simulink model "HW4_Q2"  (R2023a)
settings: Solver=FixedStepAuto  StartTime=0.0  StopTime=10.0  FixedStep=0.001  RelTol=1e-3
values from neighbouring files (symbols this model uses):
  F0 = 1    [HW4_Q2_Script.m]    (also in HW4_Q3.m)
  k = 10    [HW4_Q2_Script.m]    (also in HW4_Q3.m)
  m = 1    [HW4_Q2_Script.m]    (also in HW4_Q3.m)
settings Model: Creator=DELL  LastModifiedBy=DELL
settings SolverCC: ZeroCrossAlgorithm=Adaptive
settings DebuggingCC: IgnoredZcDiagnostic=none

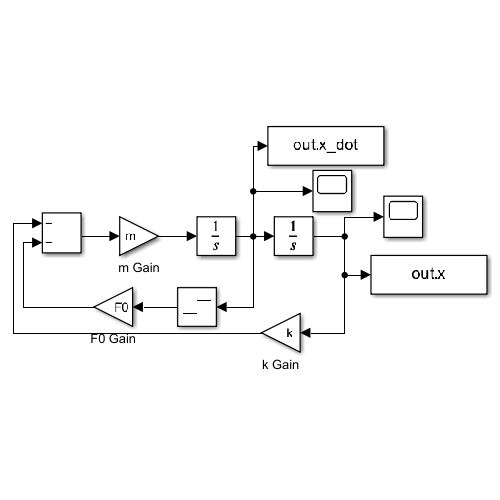
[thumbnail: Simulink's stored preview of the top-level diagram]
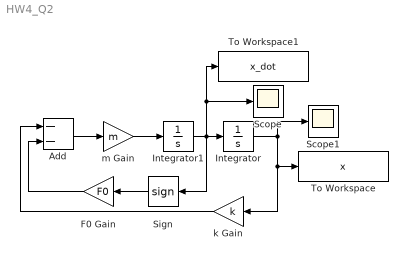
== system HW4_Q2 ==
  Add : Sum  Inputs=--
  F0 Gain : Gain  Gain=F0
  Integrator : Integrator  InitialCondition=-1
  Integrator1 : Integrator  InitialCondition=2
  Scope : Scope
  Scope1 : Scope
  Sign : Signum
  To Workspace : ToWorkspace  VariableName=x  SaveFormat=Timeseries  SampleTime=-1
  To Workspace1 : ToWorkspace  VariableName=x_dot  SaveFormat=Timeseries  SampleTime=-1
  k Gain : Gain  Gain=k
  m Gain : Gain  Gain=m
  wires:
  Integrator1/1 -> To Workspace1/1, Scope/1, Integrator/1, Sign/1
  Integrator/1 -> To Workspace/1, k Gain/1, Scope1/1
  Sign/1 -> F0 Gain/1
  Add/1 -> m Gain/1
  m Gain/1 -> Integrator1/1
  k Gain/1 -> Add/1
  F0 Gain/1 -> Add/2
